simulink subsystem "O2_dissociation"  (R2020b)
settings: Solver=VariableStepAuto  StartTime=0.0  StopTime=10.0  RelTol=1e-3
settings Model: Creator=RH  LastModifiedBy=Marco

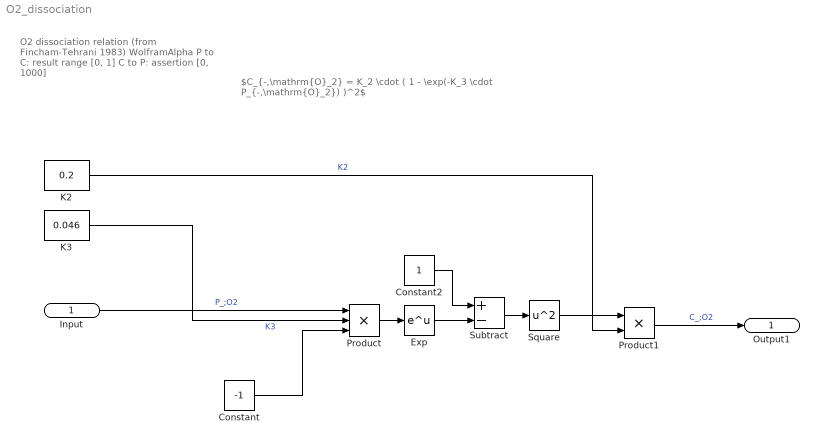
== system O2_dissociation ==
  note: O2 dissociation relation
      | (from Fincham-Tehrani 1983)
      | WolframAlpha
      |
      | P to C: result range [0, 1]
      | C to P: assertion [0, 1000]
  note: $C_{-,\mathrm{O}_2} = K_2 \cdot ( 1 - \exp(-K_3 \cdot P_{-,\mathrm{O}_2}) )^2$
  Input : Inport  Unit=mmHg
  Constant : Constant  Value=-1
  Constant2 : Constant
  Exp : Math  SaturateOnIntegerOverflow=on
  K2 : Constant  Value=0.2
  K3 : Constant  Value=0.046
  Product : Product  Inputs=3
  Product1 : Product
  Square : Math  Operator=square  SaturateOnIntegerOverflow=on
  Subtract : Sum  Inputs=+-
  Output1 : Outport  Unit=1
  wires:
  Constant/1 -> Product/3
  Product/1 -> Exp/1
  Input/1 -> Product/1  "P_;O2"
  Exp/1 -> Subtract/2
  Constant2/1 -> Subtract/1
  Subtract/1 -> Square/1
  Square/1 -> Product1/1
  K3/1 -> Product/2  "K3"
  K2/1 -> Product1/2  "K2"
  Product1/1 -> Output1/1  "C_;O2"
